simulink model "Inverters_Data_ETR07"  (R2017b)
settings: Solver=FixedStepAuto  StartTime=0.0  StopTime=10.0  RelTol=1e-3
libraries: simulink x1
settings Model: Creator=cspt  LastModifiedBy=cspt
settings RTWCC: SystemTargetFile=irt.tlc  TemplateMakefile=irt_default_tmf  Description=INTECRIO Real-Time Target
settings STFCustomTargetCC: TargetLangStandard=C99 (ISO)  UtilityFuncGeneration=Shared location  SystemTargetFile=irt.tlc
settings GRTTargetCC: UtilityFuncGeneration=Shared location  ParMdlRefBuildCompliant=off  CompOptLevelCompliant=off  ConcurrentExecutionCompliant=off  CombineOutputUpdateFcns=off  MatFileLogging=off  CPPClassGenCompliant=off  GRTInterface=on  UseToolchainInfoCompliant=off  GenerateASAP2=on

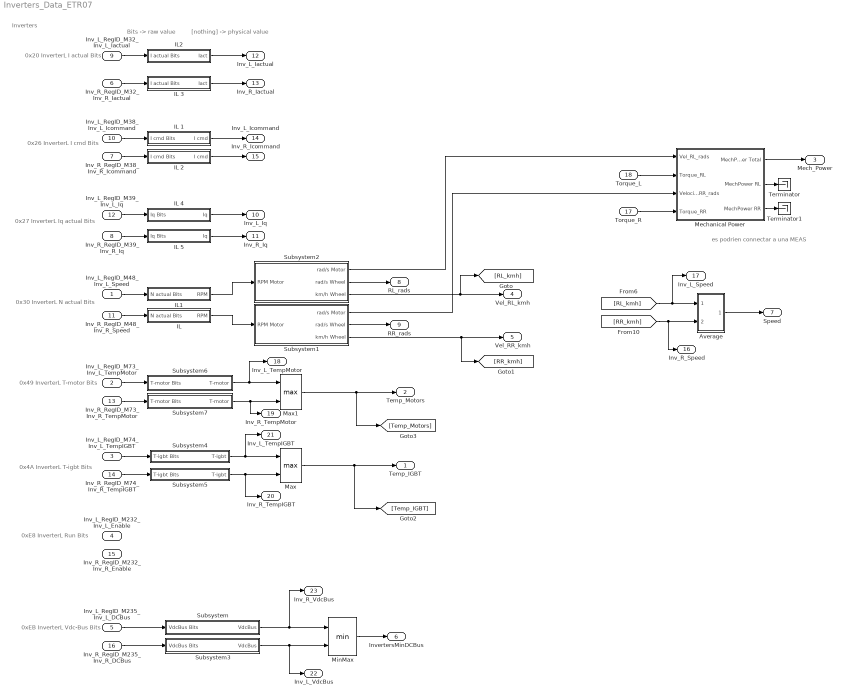
== system Inverters_Data_ETR07 ==
  note: 0x26
      | InverterL I cmd Bits
  note: Bits -> raw value
  note: 0x27
      | InverterL Iq actual Bits
  note: 0x49
      |  InverterL T-motor Bits
  note: [nothing] -> physical value
  note: 0x4A
      | InverterL T-igbt Bits
  note: 0x20
      | InverterL I actual Bits
  note: 0xEB
      | InverterL Vdc-Bus Bits
  note: 0x30
      | InverterL N actual Bits
  note: Inverters
  note: es podrien connectar a una MEAS
  note: 0xE8
      | InverterL Run Bits
  Inv_L_RegID_M48_Inv_L_Speed : Inport
  Inv_L_RegID_M73_Inv_L_TempMotor : Inport  Port=2
  Inv_L_RegID_M74_Inv_L_TempIGBT : Inport  Port=3
  Inv_L_RegID_M232_Inv_L_Enable : Inport  Port=4
  Inv_L_RegID_M235_Inv_L_DCBus : Inport  Port=5
  Inv_R_RegID_M32_Inv_R_Iactual : Inport  Port=6
  Inv_R_RegID_M38_Inv_R_Icommand : Inport  Port=7
  Inv_R_RegID_M39_Inv_R_Iq : Inport  Port=8
  Inv_L_RegID_M32_Inv_L_Iactual : Inport  Port=9
  Inv_L_RegID_M38_Inv_L_Icommand : Inport  Port=10
  Inv_R_RegID_M48_Inv_R_Speed : Inport  Port=11
  Inv_L_RegID_M39_Inv_L_Iq : Inport  Port=12
  Inv_R_RegID_M73_Inv_R_TempMotor : Inport  Port=13
  Inv_R_RegID_M74_Inv_R_TempIGBT : Inport  Port=14
  Inv_R_RegID_M232_Inv_R_Enable : Inport  Port=15
  Inv_R_RegID_M235_Inv_R_DCBus : Inport  Port=16
  Torque_R : Inport  Port=17
  Torque_L : Inport  Port=18
  Average : Subsystem
  IL : Subsystem
  IL 1 : Subsystem
  IL 2 : Subsystem
  IL 3 : Subsystem
  IL 4 : Subsystem
  IL 5 : Subsystem
  IL1 : Subsystem
  IL2 : Subsystem
  Max : MinMax  Function=max  Inputs=2
  Max1 : MinMax  Function=max  Inputs=2
  Mechanical Power : Subsystem
  MinMax : MinMax  Inputs=2
  Subsystem : Subsystem
  Subsystem1 : Subsystem
  Subsystem2 : Subsystem
  Subsystem3 : Subsystem
  Subsystem4 : Subsystem
  Subsystem5 : Subsystem
  Subsystem6 : Subsystem
  Subsystem7 : Subsystem
  Terminator : Terminator
  Terminator1 : Terminator
  Temp_IGBT : Outport
  Temp_Motors : Outport  Port=2
  Mech_Power : Outport  Port=3
  Vel_RL_kmh : Outport  Port=4
  Vel_RR_kmh : Outport  Port=5
  InvertersMinDCBus : Outport  Port=6
  Speed : Outport  Port=7
  RL_rads : Outport  Port=8
  RR_rads : Outport  Port=9
  Inv_L_Iq : Outport  Port=10
  Inv_R_Iq : Outport  Port=11
  Inv_L_Iactual : Outport  Port=12
  Inv_R_Iactual : Outport  Port=13
  Inv_L_Icommand : Outport  Port=14
  Inv_R_Icommand : Outport  Port=15
  Inv_R_Speed : Outport  Port=16
  Inv_L_Speed : Outport  Port=17
  Inv_L_TempMotor : Outport  Port=18
  Inv_R_TempMotor : Outport  Port=19
  Inv_R_TempIGBT : Outport  Port=20
  Inv_L_TempIGBT : Outport  Port=21
  Inv_L_VdcBus : Outport  Port=22
  Inv_R_VdcBus : Outport  Port=23
  wires:
  Subsystem1/2(rad/s Wheel) -> RR_rads/1
  Max1/1 -> [Temp_Motors], Temp_Motors/1
  Inv_R_RegID_M48_Inv_R_Speed/1 -> IL/1("N actual Bits ")
  Inv_R_RegID_M39_Inv_R_Iq/1 -> IL 5/1("Iq Bits ")
  [RR_kmh] -> Inv_R_Speed/1, Average/2(In2)
  Inv_L_RegID_M39_Inv_L_Iq/1 -> IL 4/1("Iq Bits ")
  Subsystem2/2(rad/s Wheel) -> RL_rads/1
  Subsystem6/1(" T-motor") -> Inv_L_TempMotor/1, Max1/1
  Subsystem2/3(km/h Wheel) -> Vel_RL_kmh/1, [RL_kmh]
  Inv_L_RegID_M48_Inv_L_Speed/1 -> IL1/1("N actual Bits ")
  Subsystem4/1(T-igbt) -> Inv_L_TempIGBT/1, Max/1
  Subsystem1/3(km/h Wheel) -> [RR_kmh], Vel_RR_kmh/1
  Torque_L/1 -> Mechanical Power/2(Torque_RL)
  Mechanical Power/3(MechPower RR) -> Terminator1/1
  Inv_L_RegID_M74_Inv_L_TempIGBT/1 -> Subsystem4/1(T-igbt Bits)
  [RL_kmh] -> Inv_L_Speed/1, Average/1(In1)
  IL1/1(RPM) -> Subsystem2/1(RPM Motor)
  Torque_R/1 -> Mechanical Power/4(Torque_RR)
  Inv_R_RegID_M73_Inv_R_TempMotor/1 -> Subsystem7/1(" T-motor Bits")
  Average/1(Out1) -> Speed/1
  Subsystem7/1(" T-motor") -> Inv_R_TempMotor/1, Max1/2
  Mechanical Power/2(MechPower RL) -> Terminator/1
  MinMax/1 -> InvertersMinDCBus/1
  Inv_L_RegID_M32_Inv_L_Iactual/1 -> IL2/1("I actual Bits ")
  Mechanical Power/1(MechPower Total) -> Mech_Power/1
  Inv_R_RegID_M38_Inv_R_Icommand/1 -> IL 2/1("I cmd Bits ")
  Inv_R_RegID_M74_Inv_R_TempIGBT/1 -> Subsystem5/1(T-igbt Bits)
  IL/1(RPM) -> Subsystem1/1(RPM Motor)
  Subsystem2/1(rad/s Motor) -> Mechanical Power/1(Vel_RL_rads)
  Max/1 -> [Temp_IGBT], Temp_IGBT/1
  Inv_L_RegID_M73_Inv_L_TempMotor/1 -> Subsystem6/1(" T-motor Bits")
  Subsystem1/1(rad/s Motor) -> Mechanical Power/3(Velocity_RR_rads)
  Inv_R_RegID_M32_Inv_R_Iactual/1 -> IL 3/1("I actual Bits ")
  Inv_L_RegID_M38_Inv_L_Icommand/1 -> IL 1/1("I cmd Bits ")
  IL 4/1(Iq) -> Inv_L_Iq/1
  IL 5/1(Iq) -> Inv_R_Iq/1
  IL 3/1(Iact) -> Inv_R_Iactual/1
  IL2/1(Iact) -> Inv_L_Iactual/1
  Subsystem5/1(T-igbt) -> Inv_R_TempIGBT/1, Max/2
  Inv_L_RegID_M235_Inv_L_DCBus/1 -> Subsystem/1(VdcBus Bits)
  Inv_R_RegID_M235_Inv_R_DCBus/1 -> Subsystem3/1(VdcBus Bits)
  Subsystem/1(VdcBus) -> Inv_R_VdcBus/1, MinMax/1
  Subsystem3/1(VdcBus) -> Inv_L_VdcBus/1, MinMax/2
  IL 2/1(I cmd) -> Inv_R_Icommand/1
  IL 1/1(I cmd) -> Inv_L_Icommand/1

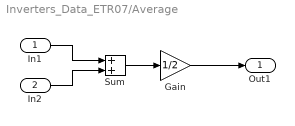
== system Inverters_Data_ETR07/Average ==
  In1 : Inport
  In2 : Inport  Port=2
  Gain : Gain  Gain=1/2
  Sum : Sum
  Out1 : Outport
  wires:
  In2/1 -> Sum/2
  Gain/1 -> Out1/1
  Sum/1 -> Gain/1
  In1/1 -> Sum/1

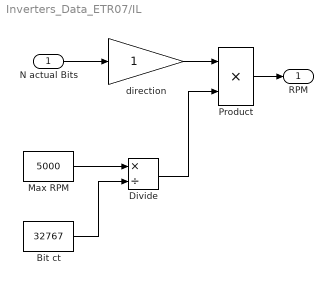
== system Inverters_Data_ETR07/IL ==
  "N actual Bits " : Inport
  Bit ct : Constant  Value=32767
  Divide : Product  Inputs=*/
  Max RPM : Constant  Value=5000
  Product : Product  OutDataTypeStr=Inherit: Inherit via back propagation
  direction : Gain
  RPM : Outport
  wires:
  Max RPM/1 -> Divide/1
  Bit ct/1 -> Divide/2
  Divide/1 -> Product/2
  "N actual Bits "/1 -> direction/1
  direction/1 -> Product/1
  Product/1 -> RPM/1

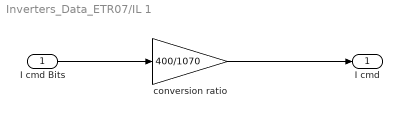
== system Inverters_Data_ETR07/IL 1 ==
  "I cmd Bits " : Inport
  conversion ratio : Gain  Gain=400/1070
  I cmd : Outport
  wires:
  "I cmd Bits "/1 -> conversion ratio/1
  conversion ratio/1 -> I cmd/1

== system Inverters_Data_ETR07/IL 2 ==
  "I cmd Bits " : Inport
  conversion ratio : Gain  Gain=400/1070
  I cmd : Outport
  wires:
  "I cmd Bits "/1 -> conversion ratio/1
  conversion ratio/1 -> I cmd/1

== system Inverters_Data_ETR07/IL 3 ==
  "I actual Bits " : Inport
  conversion ratio : Gain  Gain=400/1070
  Iact : Outport
  wires:
  "I actual Bits "/1 -> conversion ratio/1
  conversion ratio/1 -> Iact/1

== system Inverters_Data_ETR07/IL 4 ==
  "Iq Bits " : Inport
  conversion ratio : Gain  Gain=400/1070
  Iq : Outport
  wires:
  "Iq Bits "/1 -> conversion ratio/1
  conversion ratio/1 -> Iq/1

== system Inverters_Data_ETR07/IL 5 ==
  "Iq Bits " : Inport
  conversion ratio : Gain  Gain=400/1070
  Iq : Outport
  wires:
  "Iq Bits "/1 -> conversion ratio/1
  conversion ratio/1 -> Iq/1

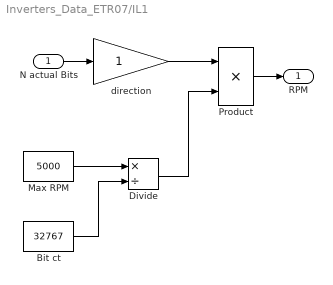
== system Inverters_Data_ETR07/IL1 ==
  "N actual Bits " : Inport
  Bit ct : Constant  Value=32767
  Divide : Product  Inputs=*/
  Max RPM : Constant  Value=5000
  Product : Product  OutDataTypeStr=Inherit: Inherit via back propagation
  direction : Gain
  RPM : Outport
  wires:
  Max RPM/1 -> Divide/1
  Bit ct/1 -> Divide/2
  Divide/1 -> Product/2
  "N actual Bits "/1 -> direction/1
  Product/1 -> RPM/1
  direction/1 -> Product/1

== system Inverters_Data_ETR07/IL2 ==
  "I actual Bits " : Inport
  conversion ratio1 : Gain  Gain=400/1070
  Iact : Outport
  wires:
  "I actual Bits "/1 -> conversion ratio1/1
  conversion ratio1/1 -> Iact/1

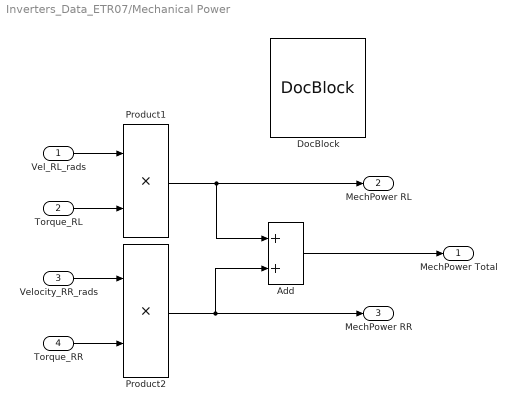
== system Inverters_Data_ETR07/Mechanical Power ==
  Vel_RL_rads : Inport
  Torque_RL : Inport  Port=2
  Velocity_RR_rads : Inport  Port=3
  Torque_RR : Inport  Port=4
  Add : Sum
  DocBlock : simulink/Model-Wide Utilities/DocBlock  DocumentType=Text
      content=|
      | This block calculates the theoretical mechanical that the motors deliver.
      |
      | The power of each motor is calculated by taking the velocity that the the inverters report and the torque that is commanded.
      | If you are a little bit of a quisquilloso you will know that the commanded torque is not the torque delivered to the motors because of the current feedback controller in the inverter.
      | A good upgrade of this module would be to read the "I actual" and do the inverse Torky to know what torque the motors are actually delivering
      |
      | Anyway.
      | Power (W) = Velocity(rad) * Torque(Nm)
      |
      | The power of each motor is reported and so is the sum of those two
  Product1 : Product
  Product2 : Product
  MechPower Total : Outport
  MechPower RL : Outport  Port=2
  MechPower RR : Outport  Port=3
  wires:
  Velocity_RR_rads/1 -> Product2/1
  Product1/1 -> MechPower RL/1, Add/1
  Vel_RL_rads/1 -> Product1/1
  Torque_RR/1 -> Product2/2
  Product2/1 -> MechPower RR/1, Add/2
  Torque_RL/1 -> Product1/2
  Add/1 -> MechPower Total/1

== system Inverters_Data_ETR07/Subsystem ==
  note: El 1.00849 es experimental
  VdcBus Bits : Inport
  Gain : Gain  Gain=1/(31.428571*1.0084926)
  VdcBus : Outport
  wires:
  VdcBus Bits/1 -> Gain/1
  Gain/1 -> VdcBus/1

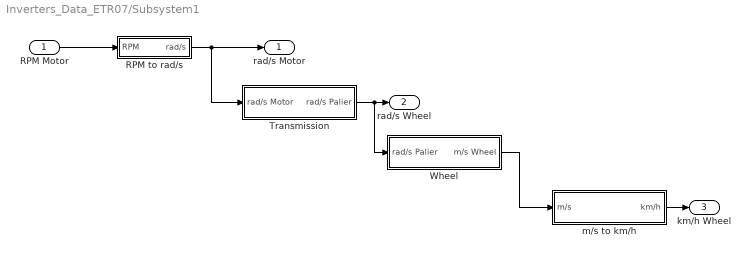
== system Inverters_Data_ETR07/Subsystem1 ==
  RPM Motor : Inport
  RPM to rad/s : Subsystem
  Transmission : Subsystem
  Wheel : Subsystem
  m/s to km/h : Subsystem
  rad/s Motor : Outport
  rad/s Wheel : Outport  Port=2
  km/h Wheel : Outport  Port=3
  wires:
  RPM Motor/1 -> RPM to rad/s/1(RPM)
  RPM to rad/s/1(rad/s) -> Transmission/1(rad/s Motor), rad/s Motor/1
  Transmission/1(rad/s Palier) -> Wheel/1(rad/s Palier), rad/s Wheel/1
  Wheel/1(m/s Wheel) -> m/s to km/h/1(m/s)
  m/s to km/h/1(km/h) -> km/h Wheel/1

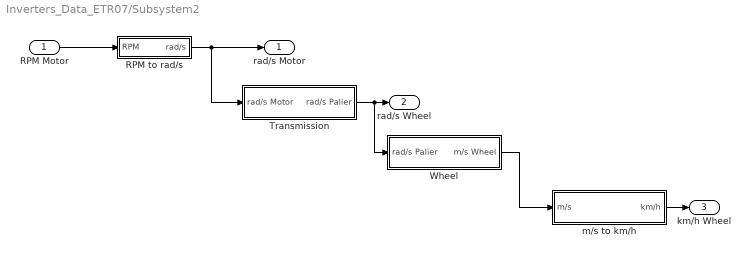
== system Inverters_Data_ETR07/Subsystem2 ==
  RPM Motor : Inport
  RPM to rad/s : Subsystem
  Transmission : Subsystem
  Wheel : Subsystem
  m/s to km/h : Subsystem
  rad/s Motor : Outport
  rad/s Wheel : Outport  Port=2
  km/h Wheel : Outport  Port=3
  wires:
  RPM Motor/1 -> RPM to rad/s/1(RPM)
  RPM to rad/s/1(rad/s) -> Transmission/1(rad/s Motor), rad/s Motor/1
  Transmission/1(rad/s Palier) -> Wheel/1(rad/s Palier), rad/s Wheel/1
  Wheel/1(m/s Wheel) -> m/s to km/h/1(m/s)
  m/s to km/h/1(km/h) -> km/h Wheel/1

== system Inverters_Data_ETR07/Subsystem3 ==
  VdcBus Bits : Inport
  Gain : Gain  Gain=1/(31.428571*1.0084926)
  VdcBus : Outport
  wires:
  VdcBus Bits/1 -> Gain/1
  Gain/1 -> VdcBus/1

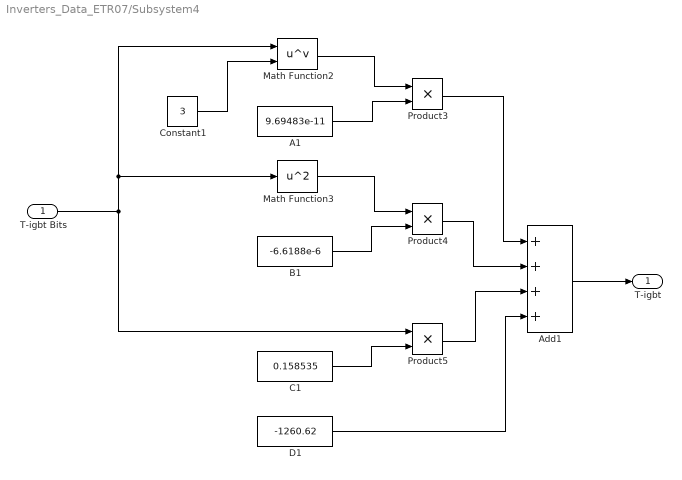
== system Inverters_Data_ETR07/Subsystem4 ==
  T-igbt Bits : Inport
  A1 : Constant  Value=9.69483e-11
  Add1 : Sum  Inputs=++++
  B1 : Constant  Value=-6.6188e-6
  C1 : Constant  Value=0.158535
  Constant1 : Constant  Value=3
  D1 : Constant  Value=-1260.62
  Math Function2 : Math  Operator=pow  SaturateOnIntegerOverflow=on
  Math Function3 : Math  Operator=square  SaturateOnIntegerOverflow=on
  Product3 : Product
  Product4 : Product
  Product5 : Product
  T-igbt : Outport
  wires:
  Constant1/1 -> Math Function2/2
  Math Function3/1 -> Product4/1
  A1/1 -> Product3/2
  B1/1 -> Product4/2
  C1/1 -> Product5/2
  Product3/1 -> Add1/1
  Math Function2/1 -> Product3/1
  T-igbt Bits/1 -> Product5/1, Math Function3/1, Math Function2/1
  D1/1 -> Add1/4
  Add1/1 -> T-igbt/1
  Product5/1 -> Add1/3
  Product4/1 -> Add1/2

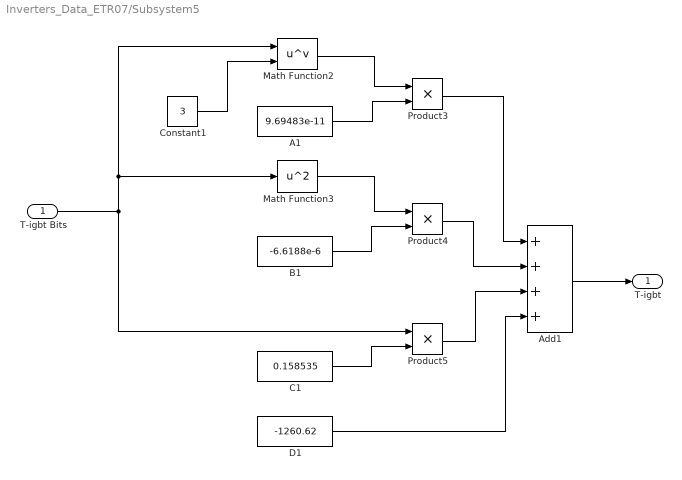
== system Inverters_Data_ETR07/Subsystem5 ==
  T-igbt Bits : Inport
  A1 : Constant  Value=9.69483e-11
  Add1 : Sum  Inputs=++++
  B1 : Constant  Value=-6.6188e-6
  C1 : Constant  Value=0.158535
  Constant1 : Constant  Value=3
  D1 : Constant  Value=-1260.62
  Math Function2 : Math  Operator=pow  SaturateOnIntegerOverflow=on
  Math Function3 : Math  Operator=square  SaturateOnIntegerOverflow=on
  Product3 : Product
  Product4 : Product
  Product5 : Product
  T-igbt : Outport
  wires:
  Constant1/1 -> Math Function2/2
  Math Function3/1 -> Product4/1
  A1/1 -> Product3/2
  B1/1 -> Product4/2
  C1/1 -> Product5/2
  Product3/1 -> Add1/1
  Math Function2/1 -> Product3/1
  T-igbt Bits/1 -> Product5/1, Math Function3/1, Math Function2/1
  D1/1 -> Add1/4
  Add1/1 -> T-igbt/1
  Product5/1 -> Add1/3
  Product4/1 -> Add1/2

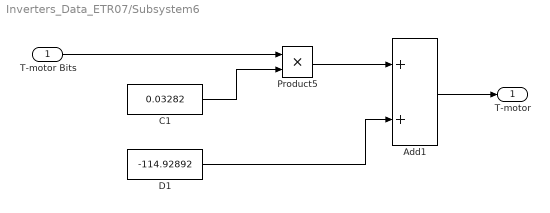
== system Inverters_Data_ETR07/Subsystem6 ==
  " T-motor Bits" : Inport
  Add1 : Sum
  C1 : Constant  Value=0.03282
  D1 : Constant  Value=-114.92892
  Product5 : Product
  " T-motor" : Outport
  wires:
  Product5/1 -> Add1/1
  D1/1 -> Add1/2
  C1/1 -> Product5/2
  Add1/1 -> " T-motor"/1
  " T-motor Bits"/1 -> Product5/1

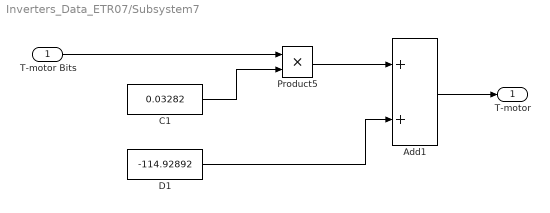
== system Inverters_Data_ETR07/Subsystem7 ==
  " T-motor Bits" : Inport
  Add1 : Sum
  C1 : Constant  Value=0.03282
  D1 : Constant  Value=-114.92892
  Product5 : Product
  " T-motor" : Outport
  wires:
  Product5/1 -> Add1/1
  D1/1 -> Add1/2
  C1/1 -> Product5/2
  Add1/1 -> " T-motor"/1
  " T-motor Bits"/1 -> Product5/1

== system Inverters_Data_ETR07/Subsystem1/RPM to rad//s ==
  RPM : Inport
  2*pi/60 : Gain  Gain=2*3.14/60
  rad/s : Outport
  wires:
  RPM/1 -> 2*pi/60/1
  2*pi/60/1 -> rad/s/1

== system Inverters_Data_ETR07/Subsystem1/Transmission ==
  rad/s Motor : Inport
  Gain : Gain  Gain=1/4
  rad/s Palier : Outport
  wires:
  rad/s Motor/1 -> Gain/1
  Gain/1 -> rad/s Palier/1

== system Inverters_Data_ETR07/Subsystem1/Wheel ==
  rad/s Palier : Inport
  Diameter [m] : Gain  Gain=0.456
  m/s Wheel : Outport
  wires:
  rad/s Palier/1 -> Diameter [m]/1
  Diameter [m]/1 -> m/s Wheel/1

== system Inverters_Data_ETR07/Subsystem1/m//s to km//h ==
  m/s : Inport
  ratio : Gain  Gain=3600/1000
  km/h : Outport
  wires:
  m/s/1 -> ratio/1
  ratio/1 -> km/h/1

== system Inverters_Data_ETR07/Subsystem2/RPM to rad//s ==
  RPM : Inport
  2*pi/60 : Gain  Gain=2*3.14/60
  rad/s : Outport
  wires:
  RPM/1 -> 2*pi/60/1
  2*pi/60/1 -> rad/s/1

== system Inverters_Data_ETR07/Subsystem2/Transmission ==
  rad/s Motor : Inport
  Gain : Gain  Gain=1/4
  rad/s Palier : Outport
  wires:
  rad/s Motor/1 -> Gain/1
  Gain/1 -> rad/s Palier/1

== system Inverters_Data_ETR07/Subsystem2/Wheel ==
  note: ESTO SE TIENE QUE CAMBIAR
  rad/s Palier : Inport
  Diameter [m] : Gain  Gain=0.457
  m/s Wheel : Outport
  wires:
  rad/s Palier/1 -> Diameter [m]/1
  Diameter [m]/1 -> m/s Wheel/1

== system Inverters_Data_ETR07/Subsystem2/m//s to km//h ==
  m/s : Inport
  ratio : Gain  Gain=3600/1000
  km/h : Outport
  wires:
  m/s/1 -> ratio/1
  ratio/1 -> km/h/1
